simulink model "MSFartoystyring2_8"  (Simulink 8.8)
settings: Solver=ode45  StartTime=tstart  StopTime=tstop  RelTol=1e-3  EnableMultiTasking=on
values from neighbouring files (symbols this model uses):
  c = 1    [run_task_2_8.m]
  K_dpsi = 2    [run_task_2_8.m]
  K_ipsi = 3    [run_task_2_8.m]
  K_iu = lambda*2    [run_task_2_8.m]
  K_ppsi = 3    [run_task_2_8.m]
  K_pu = 2*lambda    [run_task_2_8.m]
  psi0 = 150*deg2rad    (= 2.61799387799)    [run_task_2_8.m]
  r0 = 0    [run_task_2_8.m]
  tsamp = 10    [run_task_2_8.m]
  v0 = [6.63 0]'    [run_task_2_8.m]
undefined symbols (not defined in the file or in its folder): msfartoystyring
undefined symbols (not defined in the file): p0
settings Model: LogicAnalyzerSignalOrdering=6d71bc7a-7633-4ae7-a801-07df72f58b9a,e22fa85b-a01a-4f0d-8e29-b5537671e699,31bd6cee-398f-4963-ae6f-010b1011c236,fb7c025f-88bf-4fc9-b3fc-bcdb4a0b8d3c  Creator=christh  LastModifiedBy=sbuadu  ExtModeAutoUpdateStatusClock=off
settings OptimizationCC: ExpressionDepthLimit=2147483647  InitFltsAndDblsToZero=on
settings DebuggingCC: SolverPrmCheckMsg=warning

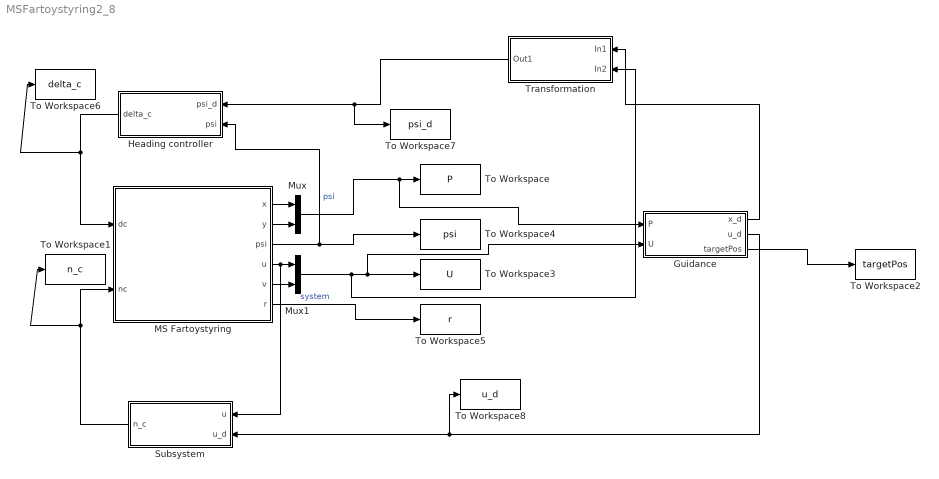
== system MSFartoystyring2_8 ==
  Guidance : Subsystem
  "Heading controller " : Subsystem
  MS Fartoystyring : Subsystem  mask(MS Fartoystyring for Assignment 3 G&C){x0=p0(1), y0=p0(2), u0=v0(1), v0=v0(2), psi0=psi0, r0=r0, c=c}
      mask prompts: x0 "x(t0) (m)"; y0 "y(t0) (m)"; u0 "u(t0) (m/s)"; v0 "v(t0) (m/s)"; psi0 "psi(t0) (rad)"; r0 "r(t0) (rad/s)"; c "current (0 or 1)"
      mask help:
      | Block corresponding to Figure 1 in the assignment text. Gives the response of the ship.
      |
      | The design speed of MS Fartoystyring is u=8.23 m/s.
      |
      | Input:
      | dc: commanded rudder (rad), dmax=25*pi/180
      | nc: commanded shaft speed (rad/s), nmax=85*2*pi/60
      |
      | Output:
      | x: north pos (m)
      | y: east pos (m)
      | u: surge (m/s)
      | v: sway (m/s)
      | psi: heading (rad)
      | r: yaw (rad/s)
      mask Help: Comments, bugs and help requests can be directed to the TA. Email on course website.
  Mux : Mux  Inputs=2
  Mux1 : Mux  Inputs=2
  Subsystem : Subsystem
  To Workspace : ToWorkspace  VariableName=P  SampleTime=tsamp
  To Workspace1 : ToWorkspace  VariableName=n_c  SampleTime=tsamp
  To Workspace2 : ToWorkspace  VariableName=targetPos  SampleTime=tsamp
  To Workspace3 : ToWorkspace  VariableName=U  SampleTime=tsamp
  To Workspace4 : ToWorkspace  VariableName=psi  SaveFormat=Timeseries  SampleTime=tsamp
  To Workspace5 : ToWorkspace  VariableName=r  SampleTime=tsamp
  To Workspace6 : ToWorkspace  VariableName=delta_c  SampleTime=tsamp
  To Workspace7 : ToWorkspace  VariableName=psi_d  SampleTime=tsamp
  To Workspace8 : ToWorkspace  VariableName=u_d  SampleTime=tsamp
  "Transformation " : Subsystem
  wires:
  MS Fartoystyring/1(x) -> Mux/1
  MS Fartoystyring/2(y) -> Mux/2
  MS Fartoystyring/4(u) -> Subsystem/1("u "), Mux1/1
  MS Fartoystyring/5(v) -> Mux1/2
  Mux/1 -> To Workspace/1, Guidance/1(P)
  Mux1/1 -> "Transformation "/2(In2), Guidance/2(U), To Workspace3/1
  MS Fartoystyring/3(psi) -> To Workspace4/1, "Heading controller "/2("psi ")  "psi"
  MS Fartoystyring/6(r) -> To Workspace5/1  "system"
  Subsystem/1("n_c ") -> To Workspace1/1, MS Fartoystyring/2(nc)
  "Heading controller "/1(delta_c) -> To Workspace6/1, MS Fartoystyring/1(dc)
  Guidance/1(x_d) -> "Transformation "/1(In1)
  Guidance/2(u_d) -> To Workspace8/1, Subsystem/2(u_d)
  Guidance/3(targetPos) -> To Workspace2/1
  "Transformation "/1(Out1) -> To Workspace7/1, "Heading controller "/1(psi_d)

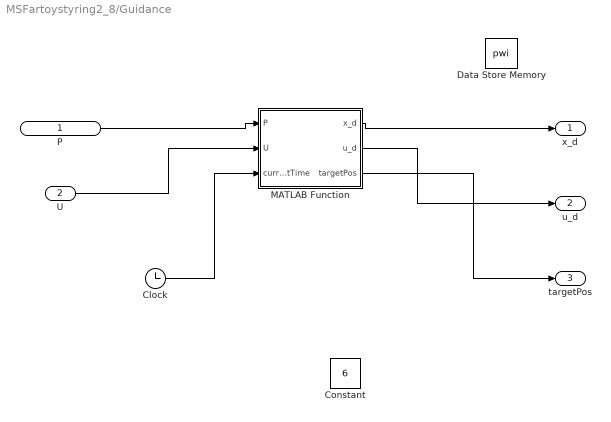
== system MSFartoystyring2_8/Guidance ==
  P : Inport
  U : Inport  Port=2
  Clock : Clock
  Constant : Constant  Value=6
  Data Store Memory : DataStoreMemory  DataStoreName=pwi  ReadBeforeWriteMsg=warning  WriteAfterWriteMsg=warning  WriteAfterReadMsg=warning  InitialValue=1  ShowAdditionalParam=off  OutDataTypeStr=double
  MATLAB Function : MATLAB Function  TreatAsAtomicUnit=on
  x_d : Outport  SampleTime=tsamp
  u_d : Outport  Port=2
  targetPos : Outport  Port=3
  wires:
  MATLAB Function/1(x_d) -> x_d/1
  P/1 -> MATLAB Function/1(P)
  U/1 -> MATLAB Function/2(U)
  Clock/1 -> MATLAB Function/3(currentTime)
  MATLAB Function/3(targetPos) -> targetPos/1
  MATLAB Function/2(u_d) -> u_d/1

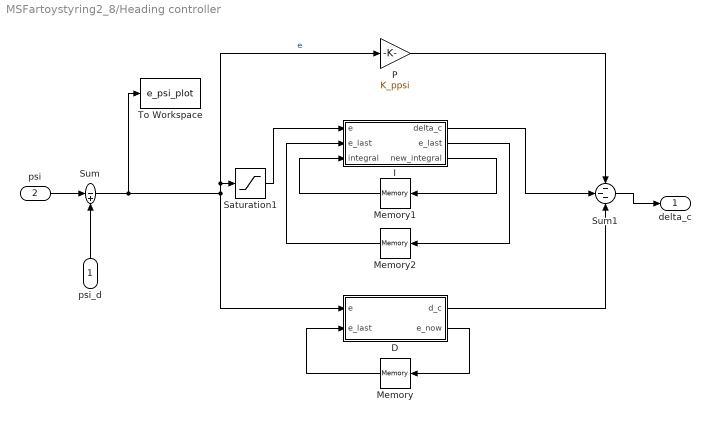
== system MSFartoystyring2_8/Heading controller  ==
  psi_d : Inport
  "psi " : Inport  Port=2
  "D " : Subsystem
  I : Subsystem
  Memory : Memory
  Memory1 : Memory
  Memory2 : Memory
  P : Gain  Gain=K_ppsi
  Saturation1 : Saturate  UpperLimit=0.05  LowerLimit=-0.05
  Sum : Sum  Inputs=|-+
  Sum1 : Sum  Inputs=---
  To Workspace : ToWorkspace  VariableName=e_psi_plot  SaveFormat=Timeseries  SampleTime=-1
  delta_c : Outport
  wires:
  "psi "/1 -> Sum/1
  psi_d/1 -> Sum/2
  Sum/1 -> To Workspace/1, Saturation1/1, P/1, "D "/1(e)  "e"
  P/1 -> Sum1/1
  Sum1/1 -> delta_c/1
  "D "/2(e_now) -> Memory/1
  Memory/1 -> "D "/2("e_last ")
  "D "/1(d_c) -> Sum1/3
  I/1(delta_c) -> Sum1/2
  I/2(e_last) -> Memory2/1
  I/3("new_integral ") -> Memory1/1
  Memory1/1 -> I/3(integral)
  Memory2/1 -> I/2("e_last ")
  Saturation1/1 -> I/1(e)

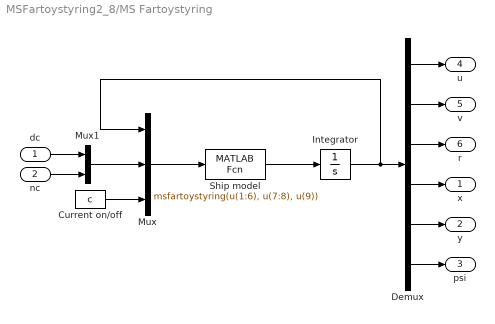
== system MSFartoystyring2_8/MS Fartoystyring ==
  dc : Inport
  nc : Inport  Port=2
  Current on/off : Constant  Value=c
  Demux : Demux  Outputs=6
  Integrator : Integrator  InitialCondition=[u0 v0 r0 x0 y0 psi0]'
  Mux : Mux  Inputs=3
  Mux1 : Mux  Inputs=2
  Ship model : MATLABFcn  MATLABFcn=msfartoystyring(u(1:6), u(7:8), u(9))  OutputDimensions=6
  x : Outport
  y : Outport  Port=2
  psi : Outport  Port=3
  u : Outport  Port=4
  v : Outport  Port=5
  r : Outport  Port=6
  wires:
  Integrator/1 -> Mux/1, Demux/1
  Mux1/1 -> Mux/2
  dc/1 -> Mux1/1
  nc/1 -> Mux1/2
  Demux/1 -> u/1
  Demux/2 -> v/1
  Demux/3 -> r/1
  Demux/4 -> x/1
  Demux/5 -> y/1
  Demux/6 -> psi/1
  Current on/off/1 -> Mux/3
  Ship model/1 -> Integrator/1
  Mux/1 -> Ship model/1

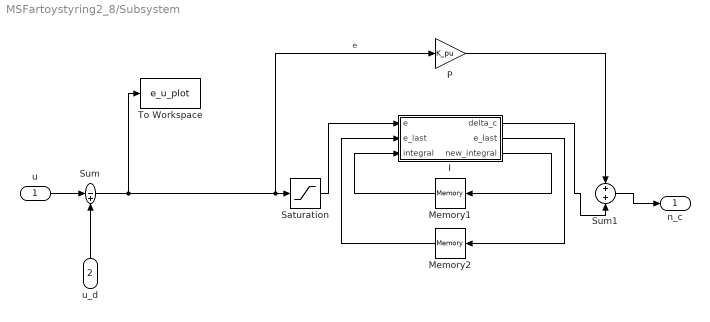
== system MSFartoystyring2_8/Subsystem ==
  "u " : Inport
  u_d : Inport  Port=2
  I : Subsystem
  Memory1 : Memory
  Memory2 : Memory
  P : Gain  Gain=K_pu
  Saturation : Saturate  UpperLimit=0.05  LowerLimit=-0.05
  Sum : Sum  Inputs=|-+
  Sum1 : Sum
  To Workspace : ToWorkspace  VariableName=e_u_plot  SaveFormat=Timeseries  SampleTime=-1
  "n_c " : Outport
  wires:
  "u "/1 -> Sum/1
  u_d/1 -> Sum/2
  Sum/1 -> To Workspace/1, Saturation/1, P/1  "e"
  P/1 -> Sum1/1
  Sum1/1 -> "n_c "/1
  I/1(delta_c) -> Sum1/2
  I/2(e_last) -> Memory2/1
  I/3("new_integral ") -> Memory1/1
  Memory1/1 -> I/3(integral)
  Memory2/1 -> I/2("e_last ")
  Saturation/1 -> I/1(e)

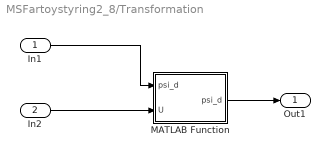
== system MSFartoystyring2_8/Transformation  ==
  In1 : Inport
  In2 : Inport  Port=2
  MATLAB Function : MATLAB Function  TreatAsAtomicUnit=on
  Out1 : Outport
  wires:
  In1/1 -> MATLAB Function/1("psi_d ")
  MATLAB Function/1(psi_d) -> Out1/1
  In2/1 -> MATLAB Function/2(U)

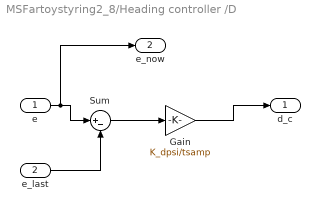
== system MSFartoystyring2_8/Heading controller /D  ==
  e : Inport
  "e_last " : Inport  Port=2
  Gain : Gain  Gain=K_dpsi/tsamp
  Sum : Sum  Inputs=|+-
  d_c : Outport
  e_now : Outport  Port=2
  wires:
  e/1 -> e_now/1, Sum/1
  "e_last "/1 -> Sum/2
  Sum/1 -> Gain/1
  Gain/1 -> d_c/1

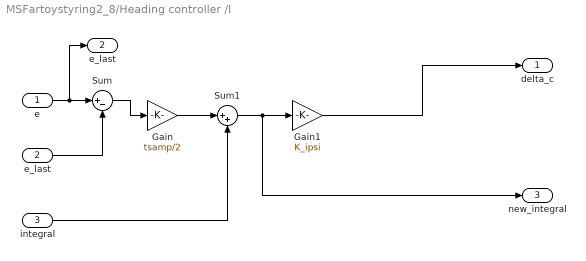
== system MSFartoystyring2_8/Heading controller /I ==
  e : Inport
  "e_last " : Inport  Port=2
  integral : Inport  Port=3
  Gain : Gain  Gain=tsamp/2
  Gain1 : Gain  Gain=K_ipsi
  Sum : Sum  Inputs=|+-
  Sum1 : Sum  Inputs=|++
  delta_c : Outport
  e_last : Outport  Port=2
  "new_integral " : Outport  Port=3
  wires:
  e/1 -> e_last/1, Sum/1
  "e_last "/1 -> Sum/2
  Sum/1 -> Gain/1
  integral/1 -> Sum1/2
  Gain/1 -> Sum1/1
  Sum1/1 -> "new_integral "/1, Gain1/1
  Gain1/1 -> delta_c/1

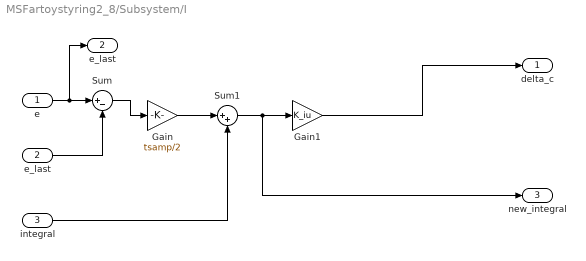
== system MSFartoystyring2_8/Subsystem/I ==
  e : Inport
  "e_last " : Inport  Port=2
  integral : Inport  Port=3
  Gain : Gain  Gain=tsamp/2
  Gain1 : Gain  Gain=K_iu
  Sum : Sum  Inputs=|+-
  Sum1 : Sum  Inputs=|++
  delta_c : Outport
  e_last : Outport  Port=2
  "new_integral " : Outport  Port=3
  wires:
  e/1 -> e_last/1, Sum/1
  "e_last "/1 -> Sum/2
  Sum/1 -> Gain/1
  integral/1 -> Sum1/2
  Gain/1 -> Sum1/1
  Sum1/1 -> "new_integral "/1, Gain1/1
  Gain1/1 -> delta_c/1

== matlab function Transformation /MATLAB Function ==
  data: psi_d input double; psi_d output double; U input double
function psi_d = fcn(psi_d, U)

u = U(1);
v = U(2);

beta = asin(v/sqrt(u^2 + v^2));
X = psi_d + atan2(v,u);
psi_d = X - beta;

end

== matlab function Guidance/MATLAB Function ==
  data: P input double; U input double; x_d output double; WP parameter double; pwi data_store_memory double; u_d output double; currentTime input double; targetPos output double
function [x_d, u_d, targetPos] = fcn(P, U, WP, currentTime)

%%
Ut = 3.0; % [m/s] Speed of the target
distance_d = 400; % [m] How far behind the target the MS Fartoystyring should track
%%


vesselPos = P';

firstWaypoint = WP(:,1)';
secondWaypoint = WP(:,2)';

% Get normalized vektor of the line
w = (secondWaypoint - firstWaypoint);
w_norm = w/norm(w);

% Get target pos
targetPos = w_norm' * Ut * currentTime + secondWaypoint';

% Distance between ships
distance = sqrt((targetPos(1)-vesselPos(1))^2 + (targetPos(2)-vesselPos(2))^2);

% Aimpoint is the targets position
aimPoint = targetPos' - (w_norm * (distance-500))*0;

% Find the angle to the aimpoint
x_d = atan2(aimPoint(2)-vesselPos(2),aimPoint(1)-vesselPos(1));

% Ensure a positive angle
if x_d < 0
    x_d = x_d + 2 * pi;
end

%% Speed guidance

distance = sqrt((targetPos(1)-vesselPos(1))^2 + (targetPos(2)-vesselPos(2))^2);
distance_e = distance-distance_d;
k = 8.9 - Ut;

speed = Ut + k * distance_e /sqrt(distance_e^2 + 2000^2);

u_d = speed; 

end
